simulink model "PRO1"  (Simulink 7.9)
settings: Solver=ode45  StartTime=0.0  StopTime=1  RelTol=1e-3
libraries: powerlib x52, powerlib_extras x1, simulink x1
settings Model: Creator=pavan  LastModifiedBy=student
settings OptimizationCC: ExpressionDepthLimit=128  InitFltsAndDblsToZero=on
settings DebuggingCC: SaveWithParameterizedLinksMsg=none  SignalResolutionControl=TryResolveAllWithWarning  MultiTaskDSMMsg=warning  MultiTaskCondExecSysMsg=none  StrictBusMsg=Warning
settings RTWCC: IncludeERTFirstTime=on
settings CodeAppCC: CustomSymbolStrType=$N$R$M_T
settings GRTTargetCC: TargetFcnLib=ansi_tfl_tmw.mat  CombineOutputUpdateFcns=off  GRTInterface=on

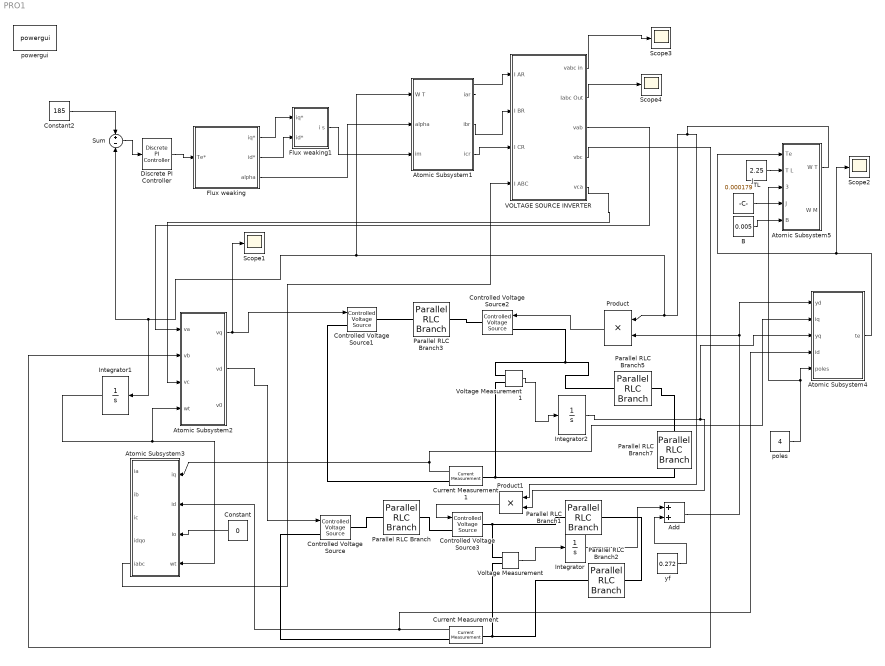
== system PRO1 ==
  Add : Sum
  Atomic Subsystem1 : Subsystem  TreatAsAtomicUnit=on
  Atomic Subsystem2 : Subsystem  TreatAsAtomicUnit=on
  Atomic Subsystem3 : Subsystem  TreatAsAtomicUnit=on
  Atomic Subsystem4 : Subsystem  TreatAsAtomicUnit=on
  Atomic Subsystem5 : Subsystem  TreatAsAtomicUnit=on
  B : Constant  Value=0.005
  Constant : Constant  Value=0
  Constant2 : Constant  Value=185
  Controlled Voltage Source{,1..3} (4 alike) : powerlib/Electrical Sources/Controlled Voltage Source  Initialize=on  Source_Type=AC  Amplitude=0  Phase=0  Frequency=0  Measurements=None
  Current Measurement : powerlib/Measurements/Current Measurement  PhasorSimulation=off  OutputType=Complex  PSBequivalent=0
  Current Measurement1 : powerlib/Measurements/Current Measurement  PhasorSimulation=off  OutputType=Complex  PSBequivalent=0
  Discrete PI Controller : powerlib_extras/Discrete  Control Blocks/Discrete PI Controller  Kp=0.3581  Ki=129.9014  Par_Limits=[1e6 -1e6]  Init=0  Ts=50e-6
  Flux weaking : Subsystem  TreatAsAtomicUnit=on
  Flux weaking1 : Subsystem  TreatAsAtomicUnit=on
  Integrator : Integrator
  Integrator1 : Integrator
  Integrator2 : Integrator
  J : Constant  Value=0.000179
  Parallel RLC Branch : powerlib/Elements/Parallel RLC Branch  LConnTagsString=a  RConnTagsString=__new0  BranchType=R  Resistance=0.8  Inductance=1e-3  SetiL0=off  InitialCurrent=0  Capacitance=1e-6  Setx0=off  InitialVoltage=0  Measurements=None
  Parallel RLC Branch{1..2,5,7} (4 alike) : powerlib/Elements/Parallel RLC Branch  LConnTagsString=a  RConnTagsString=__new0  BranchType=L  Resistance=0.8  Inductance=1e-3  SetiL0=off  InitialCurrent=0  Capacitance=1e-6  Setx0=off  InitialVoltage=0  Measurements=None
  Parallel RLC Branch3 : powerlib/Elements/Parallel RLC Branch  LConnTagsString=a  RConnTagsString=__new0  BranchType=R  Resistance=0.8  Inductance=1e-3  SetiL0=off  InitialCurrent=0  Capacitance=1e-6  Setx0=off  InitialVoltage=0  Measurements=None
  Product : Product  RndMeth=Zero
  Product1 : Product  RndMeth=Zero
  Scope{1..4} (4 alike) : Scope
      Scope1 settings: SaveName=ScopeData11
      Scope2 settings: SaveName=ScopeData2
      Scope3 settings: SaveName=ScopeData3
      Scope4 settings: SaveName=ScopeData4
  Sum : Sum  Inputs=+-
  TL : Constant  Value=2.25
  VOLTAGE SOURCE INVERTER : Subsystem  TreatAsAtomicUnit=on
      settings: ErrorFcn=-+
  Voltage Measurement : powerlib/Measurements/Voltage Measurement  PhasorSimulation=off  OutputType=Complex  PSBequivalent=0
  Voltage Measurement1 : powerlib/Measurements/Voltage Measurement  PhasorSimulation=off  OutputType=Complex  PSBequivalent=0
  poles : Constant  Value=4
  powergui : powerlib/powergui  Priority=1  SimulationMode=Continuous  SolverType=Tustin  SampleTime=50e-6  frequency=60  SPID=off  DisableSnubberDevices=off  DisableRonSwitches=off  DisableVfSwitches=off  SwTol=0  Interpol=off  DisplayEquations=off  FunctionMessages=off  frequencyindice=0  Pbase=100e6  ErrMax=1e-4  Iterations=50  UnitsV=kV  UnitsW=MW  echomessages=off  HookPort=off  EnableUseOfTLC=off  x0status=blocks  RestoreLinks=warning  ResistiveCurrentMeasurement=off  Ylog=off  Xlog=on  ShowGrid=off  save=off  variable=ZData  ZoomFFT=off  StartTime=0.0  cycles=1  DisplayStyle=1  FreqAxis=off  MaxFrequency=1000  frequencyindicesteady=1  display=off  methode=off
  yf : Constant  Value=0.272
  wires:
  Sum/1 -> Discrete PI Controller/1
  Constant2/1 -> Sum/1
  Flux weaking/3(alpha) -> Atomic Subsystem1/2("alpha\t")
  Constant/1 -> Atomic Subsystem3/3(io)
  Atomic Subsystem2/2(vd) -> Controlled Voltage Source/1
  Product/1 -> Controlled Voltage Source2/1
  Current Measurement1/1 -> Atomic Subsystem4/2(iq), Atomic Subsystem3/1(iq)
  Voltage Measurement1/1 -> Integrator2/1
  Integrator2/1 -> Atomic Subsystem4/3(yq), Product1/2
  Voltage Measurement/1 -> Integrator/1
  Integrator/1 -> Add/1
  Current Measurement/1 -> Atomic Subsystem3/2(id), Atomic Subsystem4/4(id)
  Product1/1 -> Controlled Voltage Source3/1
  Atomic Subsystem4/1(te) -> Atomic Subsystem5/1(Te), Scope2/1
  Integrator1/1 -> Atomic Subsystem3/4(wt), Atomic Subsystem2/4(wt)
  yf/1 -> Add/2
  VOLTAGE SOURCE INVERTER/1(vabc in) -> Scope3/1
  Atomic Subsystem2/1(vq) -> Scope1/1, Controlled Voltage Source1/1
  Add/1 -> Atomic Subsystem4/1(yd), Product/2
  Atomic Subsystem1/1(iar) -> VOLTAGE SOURCE INVERTER/1(I AR)
  Atomic Subsystem1/2(ibr) -> VOLTAGE SOURCE INVERTER/2(I BR)
  Atomic Subsystem3/5(iabc) -> VOLTAGE SOURCE INVERTER/4(I ABC)
  VOLTAGE SOURCE INVERTER/3(vab) -> Atomic Subsystem2/1(va)
  VOLTAGE SOURCE INVERTER/4(vbc) -> Atomic Subsystem2/2(vb)
  VOLTAGE SOURCE INVERTER/5(vca) -> Atomic Subsystem2/3(vc)
  VOLTAGE SOURCE INVERTER/2(Iabc Out) -> Scope4/1
  Discrete PI Controller/1 -> Flux weaking/1(Te*)
  Flux weaking/1(iq*) -> Flux weaking1/1(iq*)
  Flux weaking/2(id*) -> Flux weaking1/2(id*)
  Flux weaking1/1(i s) -> Atomic Subsystem1/3(im)
  Atomic Subsystem5/1(W T) -> Product1/1, Product/1, Atomic Subsystem1/1(W T), Sum/2, Integrator1/1
  poles/1 -> Atomic Subsystem5/3(POLES), Atomic Subsystem4/5(poles)
  TL/1 -> Atomic Subsystem5/2(T L)
  B/1 -> Atomic Subsystem5/5(B)
  J/1 -> Atomic Subsystem5/4(J)
  Atomic Subsystem1/3(icr) -> VOLTAGE SOURCE INVERTER/3(I CR)
  connections:
  Parallel RLC Branch/RConn1 -- Controlled Voltage Source3/LConn1
  Controlled Voltage Source3/RConn1 -- Parallel RLC Branch1/LConn1 -- Voltage Measurement/LConn1
  Parallel RLC Branch1/RConn1 -- Parallel RLC Branch2/RConn1
  Controlled Voltage Source/RConn1 -- Parallel RLC Branch/LConn1
  Current Measurement/RConn1 -- Controlled Voltage Source/LConn1
  Current Measurement/LConn1 -- Parallel RLC Branch2/LConn1 -- Voltage Measurement/LConn2
  Controlled Voltage Source1/RConn1 -- Parallel RLC Branch3/LConn1
  Parallel RLC Branch3/RConn1 -- Controlled Voltage Source2/RConn1
  Controlled Voltage Source2/LConn1 -- Parallel RLC Branch5/LConn1 -- Voltage Measurement1/LConn1
  Parallel RLC Branch7/LConn1 -- Parallel RLC Branch5/RConn1
  Current Measurement1/LConn1 -- Parallel RLC Branch7/RConn1 -- Voltage Measurement1/LConn2
  Controlled Voltage Source1/LConn1 -- Current Measurement1/RConn1

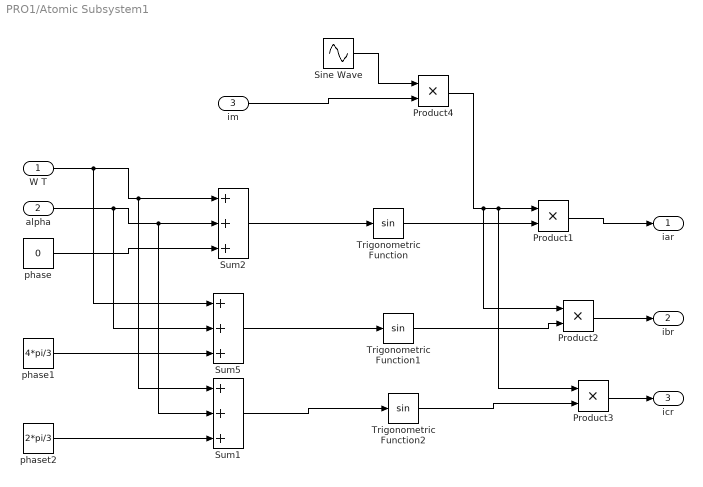
== system PRO1/Atomic Subsystem1 ==
  W T : Inport
  "alpha\t" : Inport  Port=2
  im : Inport  Port=3
  Product{1..4} (4 alike) : Product  RndMeth=Zero
  Sine Wave : Sin  SampleTime=0
  Sum1 : Sum  Inputs=+++
  Sum2 : Sum  Inputs=+++
  Sum5 : Sum  Inputs=+++
  Trigonometric Function : Trigonometry
  Trigonometric Function1 : Trigonometry
  Trigonometric Function2 : Trigonometry
  phase : Constant  Value=0
  phase1 : Constant  Value=4*pi/3
  phaset2 : Constant  Value=2*pi/3
  iar : Outport
  ibr : Outport  Port=2
  icr : Outport  Port=3
  wires:
  W T/1 -> Sum5/1, Sum2/1, Sum1/1
  "alpha\t"/1 -> Sum5/2, Sum2/2, Sum1/2
  phase/1 -> Sum2/3
  phase1/1 -> Sum5/3
  phaset2/1 -> Sum1/3
  Sum2/1 -> Trigonometric Function/1
  Sum5/1 -> Trigonometric Function1/1
  Sum1/1 -> Trigonometric Function2/1
  Trigonometric Function/1 -> Product1/2
  Sine Wave/1 -> Product4/1
  im/1 -> Product4/2
  Product4/1 -> Product2/1, Product1/1, Product3/1
  Trigonometric Function1/1 -> Product2/2
  Trigonometric Function2/1 -> Product3/2
  Product1/1 -> iar/1
  Product2/1 -> ibr/1
  Product3/1 -> icr/1

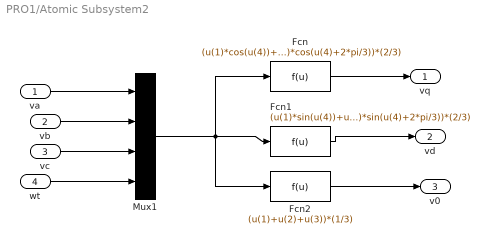
== system PRO1/Atomic Subsystem2 ==
  va : Inport
  vb : Inport  Port=2
  vc : Inport  Port=3
  wt : Inport  Port=4
  Fcn : Fcn  Expr=(u(1)*cos(u(4))+u(2)*cos(u(4)-2*pi/3)+u(3)*cos(u(4)+2*pi/3))*(2/3)
  Fcn1 : Fcn  Expr=(u(1)*sin(u(4))+u(2)*sin(u(4)-2*pi/3)+u(3)*sin(u(4)+2*pi/3))*(2/3)
  Fcn2 : Fcn  Expr=(u(1)+u(2)+u(3))*(1/3)
  Mux1 : Mux
  vq : Outport
  vd : Outport  Port=2
  v0 : Outport  Port=3
  wires:
  va/1 -> Mux1/1
  vb/1 -> Mux1/2
  vc/1 -> Mux1/3
  Mux1/1 -> Fcn1/1, Fcn/1, Fcn2/1
  Fcn1/1 -> vd/1
  Fcn2/1 -> v0/1
  Fcn/1 -> vq/1
  wt/1 -> Mux1/4

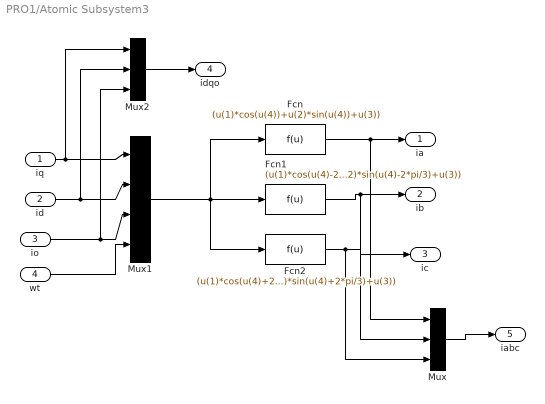
== system PRO1/Atomic Subsystem3 ==
  iq : Inport
  id : Inport  Port=2
  io : Inport  Port=3
  wt : Inport  Port=4
  Fcn : Fcn  Expr=(u(1)*cos(u(4))+u(2)*sin(u(4))+u(3))
  Fcn1 : Fcn  Expr=(u(1)*cos(u(4)-2*pi/3)+u(2)*sin(u(4)-2*pi/3)+u(3))
  Fcn2 : Fcn  Expr=(u(1)*cos(u(4)+2*pi/3)+u(2)*sin(u(4)+2*pi/3)+u(3))
  Mux : Mux  Inputs=3
      settings: DisplayOption=signals
  Mux1 : Mux
      settings: DisplayOption=signals
  Mux2 : Mux  Inputs=3
      settings: DisplayOption=signals
  ia : Outport
  ib : Outport  Port=2
  ic : Outport  Port=3
  idqo : Outport  Port=4
  iabc : Outport  Port=5
  wires:
  wt/1 -> Mux1/4
  Mux2/1 -> idqo/1
  Mux/1 -> iabc/1
  Fcn/1 -> Mux/1, ia/1
  Fcn2/1 -> Mux/3, ic/1
  Fcn1/1 -> Mux/2, ib/1
  Mux1/1 -> Fcn2/1, Fcn/1, Fcn1/1
  io/1 -> Mux2/3, Mux1/3
  id/1 -> Mux2/2, Mux1/2
  iq/1 -> Mux2/1, Mux1/1

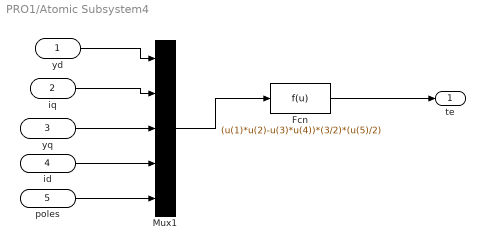
== system PRO1/Atomic Subsystem4 ==
  yd : Inport
  iq : Inport  Port=2
  yq : Inport  Port=3
  id : Inport  Port=4
  poles : Inport  Port=5
  Fcn : Fcn  Expr=(u(1)*u(2)-u(3)*u(4))*(3/2)*(u(5)/2)
  Mux1 : Mux  Inputs=5
  te : Outport
  wires:
  id/1 -> Mux1/4
  Fcn/1 -> te/1
  yq/1 -> Mux1/3
  iq/1 -> Mux1/2
  yd/1 -> Mux1/1
  Mux1/1 -> Fcn/1
  poles/1 -> Mux1/5

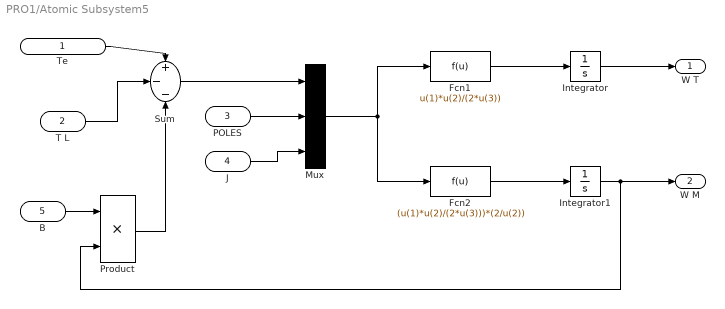
== system PRO1/Atomic Subsystem5 ==
  Te : Inport
  T L : Inport  Port=2
  POLES : Inport  Port=3
  J : Inport  Port=4
  B : Inport  Port=5
  Fcn1 : Fcn  Expr=u(1)*u(2)/(2*u(3))
  Fcn2 : Fcn  Expr=(u(1)*u(2)/(2*u(3)))*(2/u(2))
  Integrator : Integrator
  Integrator1 : Integrator
  Mux : Mux  Inputs=3
  Product : Product
  Sum : Sum  Inputs=+--
  W T : Outport
  W M : Outport  Port=2
  wires:
  T L/1 -> Sum/2
  Te/1 -> Sum/1
  Product/1 -> Sum/3
  B/1 -> Product/1
  Sum/1 -> Mux/1
  POLES/1 -> Mux/2
  J/1 -> Mux/3
  Mux/1 -> Fcn1/1, Fcn2/1
  Fcn1/1 -> Integrator/1
  Fcn2/1 -> Integrator1/1
  Integrator/1 -> W T/1
  Integrator1/1 -> W M/1, Product/2

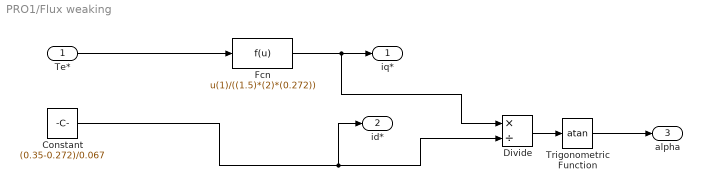
== system PRO1/Flux weaking ==
  Te* : Inport
  Constant : Constant  Value=(0.35-0.272)/0.067
  Divide : Product  Inputs=*/
  Fcn : Fcn  Expr=u(1)/((1.5)*(2)*(0.272))
  Trigonometric Function : Trigonometry  Operator=atan
  iq* : Outport
  id* : Outport  Port=2
  alpha : Outport  Port=3
  wires:
  Te*/1 -> Fcn/1
  Divide/1 -> Trigonometric Function/1
  Trigonometric Function/1 -> alpha/1
  Fcn/1 -> Divide/1, iq*/1
  Constant/1 -> id*/1, Divide/2

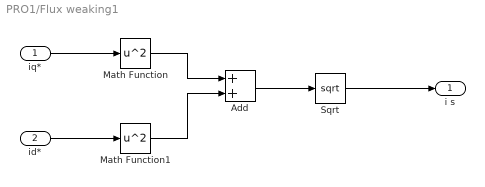
== system PRO1/Flux weaking1 ==
  iq* : Inport
  id* : Inport  Port=2
  Add : Sum
  Math Function : Math  Operator=square  SaturateOnIntegerOverflow=on
  Math Function1 : Math  Operator=square  SaturateOnIntegerOverflow=on
  Sqrt : Sqrt  SaturateOnIntegerOverflow=on
  i s : Outport
  wires:
  Add/1 -> Sqrt/1
  Sqrt/1 -> i s/1
  id*/1 -> Math Function1/1
  iq*/1 -> Math Function/1
  Math Function/1 -> Add/1
  Math Function1/1 -> Add/2

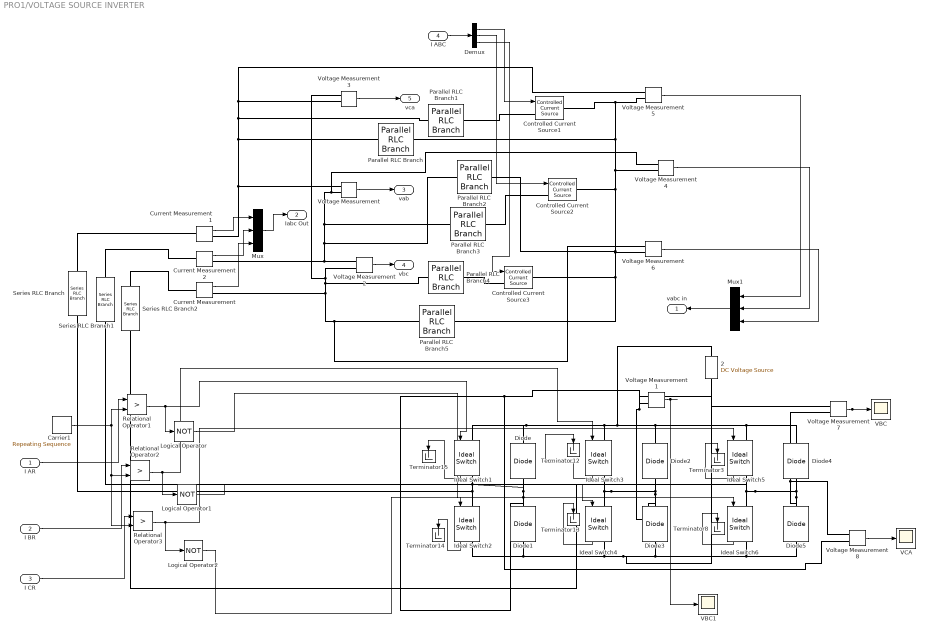
== system PRO1/VOLTAGE SOURCE INVERTER ==
  I AR : Inport
  I BR : Inport  Port=2
  I CR : Inport  Port=3
  I ABC : Inport  Port=4
  " 2" : powerlib/Electrical Sources/DC Voltage Source  Amplitude=230  Measurements=None
  Carrier1 : simulink/Sources/Repeating Sequence  rep_seq_t="[0 (1/2000)/4 (1/2000)*3/4  1/2000]"  rep_seq_y=[0 1 -1 0]
  Controlled Current Source1 : powerlib/Electrical Sources/Controlled Current Source  Initialize=on  Source_Type=AC  Amplitude=0  Phase=0  Frequency=0  Measurements=None
  Controlled Current Source2 : powerlib/Electrical Sources/Controlled Current Source  Initialize=on  Source_Type=AC  Amplitude=0  Phase=0  Frequency=0  Measurements=None
  Controlled Current Source3 : powerlib/Electrical Sources/Controlled Current Source  Initialize=on  Source_Type=AC  Amplitude=0  Phase=0  Frequency=0  Measurements=None
  Current Measurement : powerlib/Measurements/Current Measurement  PhasorSimulation=off  OutputType=Complex  PSBequivalent=0
  Current Measurement1 : powerlib/Measurements/Current Measurement  PhasorSimulation=off  OutputType=Complex  PSBequivalent=0
  Current Measurement2 : powerlib/Measurements/Current Measurement  PhasorSimulation=off  OutputType=Complex  PSBequivalent=0
  Demux : Demux  Outputs=3
  Diode{,1..5} (6 alike) : powerlib/Power Electronics/Diode  Ron=0.001  Lon=0  Vf=0.8  IC=0  UseSnubber=off  Rs=500  Cs=250e-9  Measurements=off
  Ideal Switch{1..6} (6 alike) : powerlib/Power Electronics/Ideal Switch  Ron=0.001  Lon=0  IC=0  Rs=1e5  Cs=inf  Measurements=on
  Logical Operator : Logic  Operator=NOT
  Logical Operator1 : Logic  Operator=NOT
  Logical Operator2 : Logic  Operator=NOT
  Mux : Mux  Inputs=3
  Mux1 : Mux  Inputs=3
  Parallel RLC Branch{,1..5} (6 alike) : powerlib/Elements/Parallel RLC Branch  LConnTagsString=a  RConnTagsString=__new0  BranchType=R  Resistance=1  Inductance=1e-3  SetiL0=off  InitialCurrent=0  Capacitance=1e-6  Setx0=off  InitialVoltage=0  Measurements=None
  Relational Operator1 : RelationalOperator  Operator=>  InputSameDT=on
  Relational Operator2 : RelationalOperator  Operator=>  InputSameDT=on
  Relational Operator3 : RelationalOperator  Operator=>  InputSameDT=on
  Series RLC Branch : powerlib/Elements/Series RLC Branch  LConnTagsString=__new0  RConnTagsString=__new0  BranchType=RLC  Resistance=5  Inductance=8e-3  SetiL0=off  InitialCurrent=0  Capacitance=inf  Setx0=off  InitialVoltage=0  Measurements=None
  Series RLC Branch1 : powerlib/Elements/Series RLC Branch  LConnTagsString=__new0  RConnTagsString=__new0  BranchType=RLC  Resistance=5  Inductance=8e-3  SetiL0=off  InitialCurrent=0  Capacitance=inf  Setx0=off  InitialVoltage=0  Measurements=None
  Series RLC Branch2 : powerlib/Elements/Series RLC Branch  LConnTagsString=__new0  RConnTagsString=__new0  BranchType=RLC  Resistance=5  Inductance=8e-3  SetiL0=off  InitialCurrent=0  Capacitance=inf  Setx0=off  InitialVoltage=0  Measurements=None
  Terminator{3,8,12..15} (6 alike) : Terminator
  VBC : Scope
  VBC1 : Scope
      settings: SaveName=ScopeData7
  VCA : Scope
      settings: SaveName=ScopeData8
  Voltage Measurement{,1..8} (9 alike) : powerlib/Measurements/Voltage Measurement  PhasorSimulation=off  OutputType=Complex  PSBequivalent=0
  vabc in : Outport
  Iabc Out : Outport  Port=2
  vab : Outport  Port=3
  vbc : Outport  Port=4
  vca : Outport  Port=5
  wires:
  Current Measurement1/1 -> Mux/1
  Current Measurement2/1 -> Mux/2
  Current Measurement/1 -> Mux/3
  Mux/1 -> Iabc Out/1
  Voltage Measurement3/1 -> vca/1
  Voltage Measurement/1 -> vab/1
  Voltage Measurement2/1 -> vbc/1
  Voltage Measurement5/1 -> Mux1/1
  Voltage Measurement4/1 -> Mux1/2
  Voltage Measurement6/1 -> Mux1/3
  Demux/1 -> Controlled Current Source1/1
  Demux/3 -> Controlled Current Source3/1
  Demux/2 -> Controlled Current Source2/1
  Relational Operator1/1 -> Logical Operator/1, Ideal Switch1/1
  Relational Operator2/1 -> Logical Operator1/1, Ideal Switch3/1
  Relational Operator3/1 -> Logical Operator2/1, Ideal Switch5/1
  Logical Operator/1 -> Ideal Switch2/1
  Logical Operator1/1 -> Ideal Switch4/1
  Logical Operator2/1 -> Ideal Switch6/1
  Carrier1/1 -> Relational Operator2/2, Relational Operator3/2, Relational Operator1/2
  I CR/1 -> Relational Operator3/1
  I BR/1 -> Relational Operator2/1
  I AR/1 -> Relational Operator1/1
  I ABC/1 -> Demux/1
  Ideal Switch5/1 -> Terminator3/1
  Ideal Switch6/1 -> Terminator8/1
  Ideal Switch3/1 -> Terminator12/1
  Ideal Switch4/1 -> Terminator13/1
  Ideal Switch2/1 -> Terminator14/1
  Ideal Switch1/1 -> Terminator15/1
  Voltage Measurement1/1 -> VBC1/1
  Voltage Measurement7/1 -> VBC/1
  Voltage Measurement8/1 -> VCA/1
  Mux1/1 -> vabc in/1
  connections:
  Controlled Current Source1/RConn1 -- Parallel RLC Branch/RConn1 -- Parallel RLC Branch2/RConn1 -- Controlled Current Source3/RConn1 -- Parallel RLC Branch5/RConn1 -- Voltage Measurement6/LConn2 -- Controlled Current Source2/RConn1 -- Voltage Measurement4/LConn2 -- Voltage Measurement5/LConn2
  Current Measurement/RConn1 -- Parallel RLC Branch4/LConn1 -- Voltage Measurement3/LConn1 -- Voltage Measurement2/LConn2 -- Voltage Measurement6/LConn1 -- Parallel RLC Branch5/LConn1
  Voltage Measurement/LConn2 -- Voltage Measurement4/LConn1 -- Parallel RLC Branch2/LConn1 -- Current Measurement2/RConn1 -- Voltage Measurement2/LConn1 -- Parallel RLC Branch3/LConn1
  Current Measurement1/RConn1 -- Parallel RLC Branch/LConn1 -- Parallel RLC Branch1/LConn1 -- Voltage Measurement3/LConn2 -- Voltage Measurement5/LConn1 -- Voltage Measurement/LConn1
  Parallel RLC Branch1/RConn1 -- Controlled Current Source1/LConn1
  Parallel RLC Branch4/RConn1 -- Controlled Current Source3/LConn1
  Parallel RLC Branch3/RConn1 -- Controlled Current Source2/LConn1
  Ideal Switch2/LConn1 -- Ideal Switch1/RConn1 -- Diode/LConn1 -- Diode1/RConn1 -- Voltage Measurement8/LConn2 -- Voltage Measurement1/LConn1 -- Series RLC Branch/LConn1
  Ideal Switch3/LConn1 -- Diode/RConn1 -- Ideal Switch1/LConn1 -- Diode2/RConn1 -- Diode4/RConn1 -- Ideal Switch5/LConn1 -- " 2"/RConn1
  Ideal Switch4/RConn1 -- Ideal Switch2/RConn1 -- Diode1/LConn1 -- Diode3/LConn1 -- Diode5/LConn1 -- Ideal Switch6/RConn1 -- " 2"/LConn1
  Ideal Switch4/LConn1 -- Ideal Switch3/RConn1 -- Diode2/LConn1 -- Diode3/RConn1 -- Voltage Measurement1/LConn2 -- Voltage Measurement7/LConn1 -- Series RLC Branch1/LConn1
  Ideal Switch5/RConn1 -- Ideal Switch6/LConn1 -- Diode4/LConn1 -- Diode5/RConn1 -- Voltage Measurement8/LConn1 -- Voltage Measurement7/LConn2 -- Series RLC Branch2/LConn1
  Series RLC Branch/RConn1 -- Current Measurement1/LConn1
  Series RLC Branch1/RConn1 -- Current Measurement2/LConn1
  Series RLC Branch2/RConn1 -- Current Measurement/LConn1
